simulink model "Static_pFIR"  (R2019b)
settings: Solver=FixedStepAuto  StartTime=0.0  StopTime=stop_time  RelTol=1e-3  EnableMultiTasking=on
InitFcn:
  | sm_callback_init
undefined symbols (not defined in the file or in its folder): a, b, B_k_0_init, c, FIR_0_Size, FIR_0_Uprate, Ts
libraries: simulink x10, hdlsllib x2
settings Model: Creator=Balad  LastModifiedBy=cb54103
settings DataIOCC: SaveOutput=off  SaveTime=off
settings OptimizationCC: BlockReduction=off  ConditionallyExecuteInputs=off  DefaultParameterBehavior=Inlined
settings DebuggingCC: SingleTaskRateTransMsg=error
settings SFSimCC: CustomCodeUndefinedFunction=UseInterfaceOnly

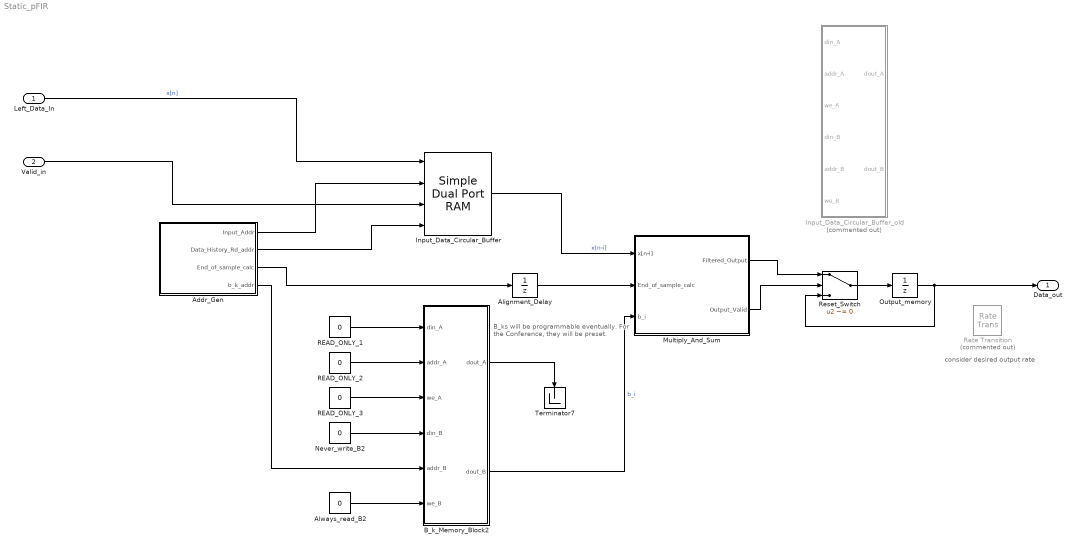
== system Static_pFIR ==
  note: consider desired output rate
  note: B_ks will be programmable eventually.
      | For the Conference, they will be preset.
  Left_Data_In : Inport  OutDataTypeStr=fixdt(1,32,28)  PortDimensions=[1 1]  SampleTime=[2.0345052083333333e-08,0]
  Valid_in : Inport  Port=2  OutDataTypeStr=boolean  PortDimensions=[1 1]  SampleTime=[2.0345052083333333e-08,0]
  "Addr_Gen " : Subsystem
  Alignment_Delay : UnitDelay  SampleTime=-1  HasFrameUpgradeWarning=on
  Always_read_B2 : Constant  Value=0  OutDataTypeStr=boolean  SampleTime=Ts/FIR_0_Uprate
  B_k_Memory_Block2 : Subsystem  AncestorBlock=DualPortRam_UNLOCKED/Dual Rate Dual Port RAM1  mask(Dual-rate dual-port RAM){ram_size=FIR_0_Size}
      mask prompts: ram_size "Address port width (2 to 28 bits)"
      mask help: This block simulates a dual-clock dual-port RAM with two data output ports.
      mask init:
      | hdlblkmask_drdpram();
      mask Help: helpview([docroot '/simulink/helptargets.map'],'HDL_dual_rate_dual_port_ram');
  Input_Data_Circular_Buffer : hdlsllib/HDL RAMs/Simple Dual Port RAM  ram_size=FIR_0_Size
      settings: SourceProductName=Simulink  SourceProductBaseCode=SL
  Input_Data_Circular_Buffer_old : Subsystem  Commented=on  AncestorBlock=DualPortRam_UNLOCKED/Dual Rate Dual Port RAM1  mask(Dual-rate dual-port RAM){ram_size=FIR_0_Size}
      mask prompts: ram_size "Address port width (2 to 28 bits)"
      mask help: This block simulates a dual-clock dual-port RAM with two data output ports.
      mask init:
      | hdlblkmask_drdpram();
      mask Help: helpview([docroot '/simulink/helptargets.map'],'HDL_dual_rate_dual_port_ram');
  Multiply_And_Sum : Subsystem
  Never_write_B2 : Constant  Value=0  OutDataTypeStr=fixdt(1,W_bits, F_bits)  SampleTime=Ts/FIR_0_Uprate
  Output_memory : UnitDelay  SampleTime=-1  HasFrameUpgradeWarning=on
  READ_ONLY_1 : Constant  Value=0  OutDataTypeStr=fixdt(1,W_bits, F_bits)  SampleTime=Ts/FIR_0_Uprate
  READ_ONLY_2 : Constant  Value=0  OutDataTypeStr=fixdt(0,FIR_0_Size, 0)  SampleTime=Ts/FIR_0_Uprate
  READ_ONLY_3 : Constant  Value=0  OutDataTypeStr=boolean  SampleTime=Ts/FIR_0_Uprate
  Rate Transition : RateTransition  Commented=on  OutPortSampleTime=Ts
  Reset_Switch : Switch  Criteria=u2 ~= 0
  Terminator7 : Terminator
  Data_out : Outport  OutDataTypeStr=fixdt(1,32,28)  PortDimensions=1  SampleTime=[2.0345052083333333e-08,0]  VectorParamsAs1DForOutWhenUnconnected=off
  wires:
  READ_ONLY_2/1 -> B_k_Memory_Block2/2(addr_A)
  Always_read_B2/1 -> B_k_Memory_Block2/6(we_B)
  B_k_Memory_Block2/1(dout_A) -> Terminator7/1
  "Addr_Gen "/3(End_of_sample_calc) -> Alignment_Delay/1
  B_k_Memory_Block2/2(dout_B) -> Multiply_And_Sum/3(b_i)  "b_i"
  Reset_Switch/1 -> Output_memory/1
  Multiply_And_Sum/2(Output_Valid) -> Reset_Switch/2
  READ_ONLY_1/1 -> B_k_Memory_Block2/1(din_A)
  Never_write_B2/1 -> B_k_Memory_Block2/4(din_B)
  Input_Data_Circular_Buffer/1 -> Multiply_And_Sum/1(x[n-i])  "x[n-i]"
  "Addr_Gen "/2(Data_History_Rd_addr) -> Input_Data_Circular_Buffer/4
  Valid_in/1 -> Input_Data_Circular_Buffer/3
  Output_memory/1 -> Reset_Switch/3, Data_out/1
  READ_ONLY_3/1 -> B_k_Memory_Block2/3(we_A)
  "Addr_Gen "/1(Input_Addr) -> Input_Data_Circular_Buffer/2
  Multiply_And_Sum/1(Filtered_Output) -> Reset_Switch/1
  "Addr_Gen "/4(b_k_addr) -> B_k_Memory_Block2/5(addr_B)
  Left_Data_In/1 -> Input_Data_Circular_Buffer/1  "x[n]"
  Alignment_Delay/1 -> Multiply_And_Sum/2(End_of_sample_calc)

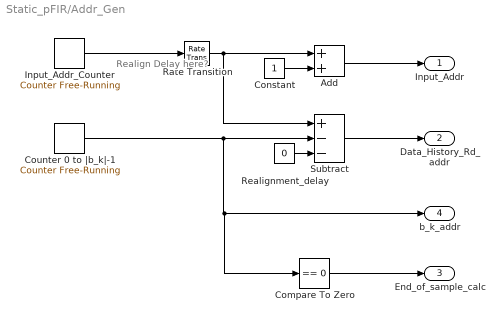
== system Static_pFIR/Addr_Gen  ==
  note: Realign Delay here?
  Add : Sum  OutDataTypeStr=Inherit: Same as first input
  Compare To Zero : simulink/Logic and Bit Operations/Compare To Zero  relop===  OutDataTypeStr=boolean  ZeroCross=off
  Constant : Constant  OutDataTypeStr=fixdt(0, FIR_0_Size,0)  SampleTime=-1
  Counter 0 to |b_k|-1 : simulink/Sources/Counter Free-Running  NumBits=FIR_0_Size  tsamp=Ts/FIR_0_Uprate
  Input_Addr_Counter : simulink/Sources/Counter Free-Running  NumBits=FIR_0_Size  tsamp=Ts
  Rate Transition : RateTransition  OutPortSampleTime=Ts/FIR_0_Uprate
  Realignment_delay : Constant  Value=0  OutDataTypeStr=fixdt(0, FIR_0_Size,0)  SampleTime=-1
  Subtract : Sum  Inputs=+--  OutDataTypeStr=Inherit: Same as first input
  Input_Addr : Outport  VectorParamsAs1DForOutWhenUnconnected=off
  Data_History_Rd_addr : Outport  Port=2  VectorParamsAs1DForOutWhenUnconnected=off
  End_of_sample_calc : Outport  Port=3  VectorParamsAs1DForOutWhenUnconnected=off
  b_k_addr : Outport  Port=4  VectorParamsAs1DForOutWhenUnconnected=off
  wires:
  Rate Transition/1 -> Add/1, Subtract/1
  Compare To Zero/1 -> End_of_sample_calc/1
  Realignment_delay/1 -> Subtract/3
  Constant/1 -> Add/2
  Add/1 -> Input_Addr/1
  Input_Addr_Counter/1 -> Rate Transition/1
  Subtract/1 -> Data_History_Rd_addr/1
  Counter 0 to |b_k|-1/1 -> b_k_addr/1, Compare To Zero/1, Subtract/2

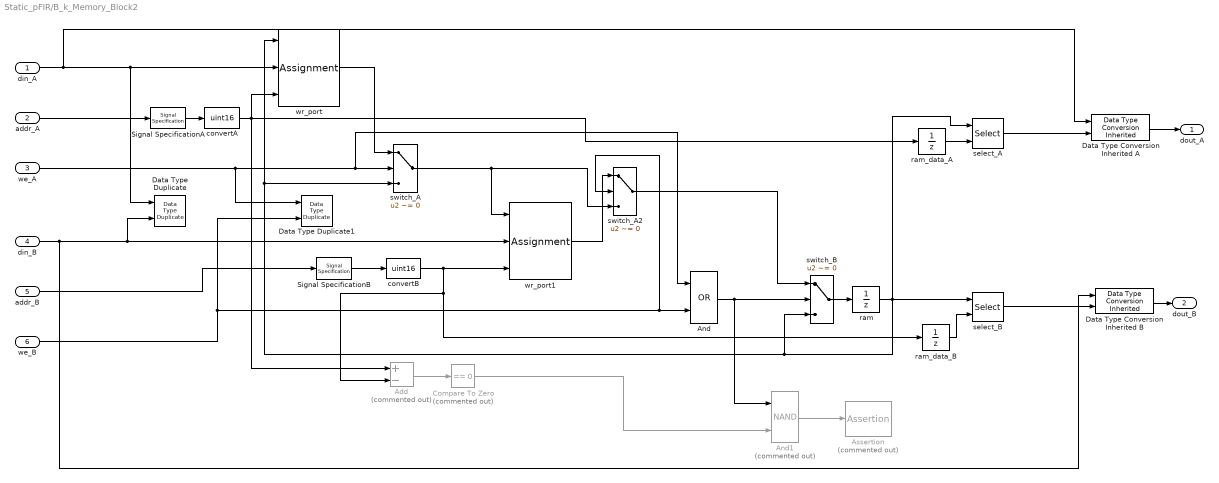
== system Static_pFIR/B_k_Memory_Block2 ==
  din_A : Inport
  addr_A : Inport  Port=2
  we_A : Inport  Port=3  OutDataTypeStr=boolean
  din_B : Inport  Port=4
  addr_B : Inport  Port=5
  we_B : Inport  Port=6  OutDataTypeStr=boolean
  Add : Sum  Commented=on  Inputs=+-
  And : Logic  Operator=OR  AllPortsSameDT=off  OutDataTypeStr=boolean
  And1 : Logic  Commented=on  Operator=NAND  AllPortsSameDT=off  OutDataTypeStr=boolean
  Assertion : Assertion  Commented=on  StopWhenAssertionFail=off
  Compare To Zero : simulink/Logic and Bit Operations/Compare To Zero  Commented=on  relop===  OutDataTypeStr=boolean
  Data Type Conversion Inherited A : simulink/Signal Attributes/Data Type Conversion Inherited  ConvertRealWorld=Real World Value  DoSatur=off
      settings: SourceProductName=Simulink  SourceProductBaseCode=SL
  Data Type Conversion Inherited B : simulink/Signal Attributes/Data Type Conversion Inherited  ConvertRealWorld=Real World Value  DoSatur=off
      settings: SourceProductName=Simulink  SourceProductBaseCode=SL
  Data Type Duplicate : DataTypeDuplicate
  Data Type Duplicate1 : DataTypeDuplicate
  Signal SpecificationA : SignalSpecification  OutDataTypeStr=fixdt(0,ram_size,0)  Dimensions=1
  Signal SpecificationB : SignalSpecification  OutDataTypeStr=fixdt(0,ram_size,0)  Dimensions=1
  convertA : DataTypeConversion  OutDataTypeStr=uint16
  convertB : DataTypeConversion  OutDataTypeStr=uint16
  ram : UnitDelay  InitialCondition=B_k_0_init  SampleTime=-1  HasFrameUpgradeWarning=on
  ram_data_A : UnitDelay  SampleTime=-1  HasFrameUpgradeWarning=on
  ram_data_B : UnitDelay  SampleTime=-1  HasFrameUpgradeWarning=on
  select_A : Selector  IndexMode=Zero-based  InputPortWidth=2^ram_size  IndexOptions=Index vector (port)  Indices=[1 3]  OutputSizes=1
  select_B : Selector  IndexMode=Zero-based  InputPortWidth=2^ram_size  IndexOptions=Index vector (port)  Indices=[1 3]  OutputSizes=1
  switch_A : Switch  Criteria=u2 ~= 0
  switch_A2 : Switch  Criteria=u2 ~= 0
  switch_B : Switch  Criteria=u2 ~= 0
  wr_port : Assignment  IndexMode=Zero-based  IndexOptions=Index vector (port)  Indices=1  OutputSizes=[1 1]
  wr_port1 : Assignment  IndexMode=Zero-based  IndexOptions=Index vector (port)  Indices=1  OutputSizes=[1 1]
  dout_A : Outport  VectorParamsAs1DForOutWhenUnconnected=off
  dout_B : Outport  Port=2  VectorParamsAs1DForOutWhenUnconnected=off
  wires:
  Data Type Conversion Inherited A/1 -> dout_A/1
  select_A/1 -> Data Type Conversion Inherited A/2
  Data Type Conversion Inherited B/1 -> dout_B/1
  select_B/1 -> Data Type Conversion Inherited B/2
  addr_A/1 -> Signal SpecificationA/1
  din_B/1 -> Data Type Conversion Inherited B/1, Data Type Duplicate/2, wr_port1/2
  convertB/1 -> wr_port1/3, Add/2, ram_data_B/1
  din_A/1 -> Data Type Conversion Inherited A/1, wr_port/2, Data Type Duplicate/1
  ram_data_A/1 -> select_A/2
  we_A/1 -> switch_A/2, And/1, Data Type Duplicate1/1
  ram_data_B/1 -> select_B/2
  addr_B/1 -> Signal SpecificationB/1
  switch_A/1 -> switch_A2/3, wr_port1/1
  we_B/1 -> Data Type Duplicate1/2, And/2, switch_A2/2
  Compare To Zero/1 -> And1/2
  Add/1 -> Compare To Zero/1
  wr_port1/1 -> switch_A2/1
  And/1 -> switch_B/2, And1/1
  wr_port/1 -> switch_A/1
  ram/1 -> select_A/1, wr_port/1, switch_A/3, switch_B/3, select_B/1
  convertA/1 -> Add/1, wr_port/3, ram_data_A/1
  switch_B/1 -> ram/1
  Signal SpecificationB/1 -> convertB/1
  Signal SpecificationA/1 -> convertA/1
  And1/1 -> Assertion/1
  switch_A2/1 -> switch_B/1

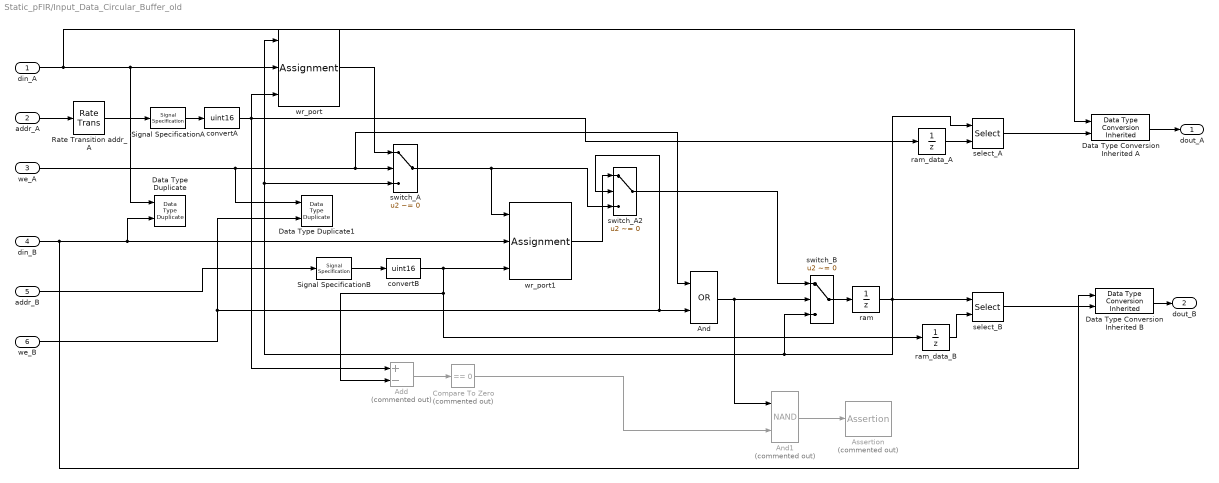
== system Static_pFIR/Input_Data_Circular_Buffer_old ==
  din_A : Inport
  addr_A : Inport  Port=2
  we_A : Inport  Port=3  OutDataTypeStr=boolean
  din_B : Inport  Port=4
  addr_B : Inport  Port=5
  we_B : Inport  Port=6  OutDataTypeStr=boolean
  Add : Sum  Commented=on  Inputs=+-
  And : Logic  Operator=OR  AllPortsSameDT=off  OutDataTypeStr=boolean
  And1 : Logic  Commented=on  Operator=NAND  AllPortsSameDT=off  OutDataTypeStr=boolean
  Assertion : Assertion  Commented=on  StopWhenAssertionFail=off
  Compare To Zero : simulink/Logic and Bit Operations/Compare To Zero  Commented=on  relop===  OutDataTypeStr=boolean
  Data Type Conversion Inherited A : simulink/Signal Attributes/Data Type Conversion Inherited  ConvertRealWorld=Real World Value  DoSatur=off
      settings: SourceProductName=Simulink  SourceProductBaseCode=SL
  Data Type Conversion Inherited B : simulink/Signal Attributes/Data Type Conversion Inherited  ConvertRealWorld=Real World Value  DoSatur=off
      settings: SourceProductName=Simulink  SourceProductBaseCode=SL
  Data Type Duplicate : DataTypeDuplicate
  Data Type Duplicate1 : DataTypeDuplicate
  Rate Transition addr_A : RateTransition
  Signal SpecificationA : SignalSpecification  OutDataTypeStr=fixdt(0,ram_size,0)  Dimensions=1
  Signal SpecificationB : SignalSpecification  OutDataTypeStr=fixdt(0,ram_size,0)  Dimensions=1
  convertA : DataTypeConversion  OutDataTypeStr=uint16
  convertB : DataTypeConversion  OutDataTypeStr=uint16
  ram : UnitDelay  SampleTime=-1  HasFrameUpgradeWarning=on
  ram_data_A : UnitDelay  SampleTime=-1  HasFrameUpgradeWarning=on
  ram_data_B : UnitDelay  SampleTime=-1  HasFrameUpgradeWarning=on
  select_A : Selector  IndexMode=Zero-based  InputPortWidth=2^ram_size  IndexOptions=Index vector (port)  Indices=[1 3]  OutputSizes=1
  select_B : Selector  IndexMode=Zero-based  InputPortWidth=2^ram_size  IndexOptions=Index vector (port)  Indices=[1 3]  OutputSizes=1
  switch_A : Switch  Criteria=u2 ~= 0
  switch_A2 : Switch  Criteria=u2 ~= 0
  switch_B : Switch  Criteria=u2 ~= 0
  wr_port : Assignment  IndexMode=Zero-based  IndexOptions=Index vector (port)  Indices=1  OutputSizes=[1 1]
  wr_port1 : Assignment  IndexMode=Zero-based  IndexOptions=Index vector (port)  Indices=1  OutputSizes=[1 1]
  dout_A : Outport  VectorParamsAs1DForOutWhenUnconnected=off
  dout_B : Outport  Port=2  VectorParamsAs1DForOutWhenUnconnected=off
  wires:
  switch_A2/1 -> switch_B/1
  And1/1 -> Assertion/1
  Signal SpecificationA/1 -> convertA/1
  Signal SpecificationB/1 -> convertB/1
  switch_B/1 -> ram/1
  convertA/1 -> ram_data_A/1, wr_port/3, Add/1
  ram/1 -> select_B/1, switch_B/3, switch_A/3, wr_port/1, select_A/1
  wr_port/1 -> switch_A/1
  And/1 -> And1/1, switch_B/2
  wr_port1/1 -> switch_A2/1
  Add/1 -> Compare To Zero/1
  Compare To Zero/1 -> And1/2
  we_B/1 -> switch_A2/2, And/2, Data Type Duplicate1/2
  switch_A/1 -> wr_port1/1, switch_A2/3
  addr_B/1 -> Signal SpecificationB/1
  ram_data_B/1 -> select_B/2
  we_A/1 -> Data Type Duplicate1/1, And/1, switch_A/2
  ram_data_A/1 -> select_A/2
  din_A/1 -> Data Type Conversion Inherited A/1, Data Type Duplicate/1, wr_port/2
  convertB/1 -> ram_data_B/1, Add/2, wr_port1/3
  din_B/1 -> Data Type Conversion Inherited B/1, wr_port1/2, Data Type Duplicate/2
  addr_A/1 -> Rate Transition addr_A/1
  Rate Transition addr_A/1 -> Signal SpecificationA/1
  select_B/1 -> Data Type Conversion Inherited B/2
  Data Type Conversion Inherited B/1 -> dout_B/1
  select_A/1 -> Data Type Conversion Inherited A/2
  Data Type Conversion Inherited A/1 -> dout_A/1

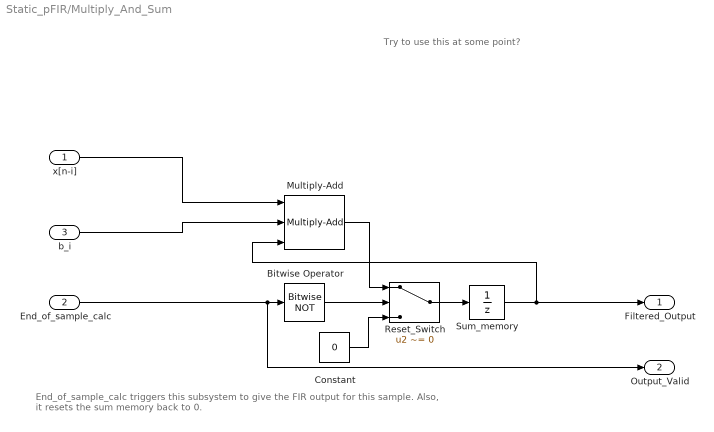
== system Static_pFIR/Multiply_And_Sum ==
  note: End_of_sample_calc triggers this subsystem to give the FIR output for this sample.
      | Also, it resets the sum memory back to 0.
  note: Try to use this at some point?
  x[n-i] : Inport
  End_of_sample_calc : Inport  Port=2
  b_i : Inport  Port=3
  Bitwise Operator : simulink/Logic and Bit Operations/Bitwise Operator  logicop=NOT  UseBitMask=off  BitMask=bin2dec('11011001')  BitMaskRealWorld=Stored Integer
  Constant : Constant  Value=0  OutDataTypeStr=fixdt(1, W_bits, F_bits)  SampleTime=Ts/FIR_0_Uprate
  Multiply-Add : hdlsllib/HDL Operations/Multiply-Add  Function=c+(a.*b)  datatype=Inherit: Same as first input  DoSatur=off  FMA=off
      settings: SourceProductName=Simulink  SourceProductBaseCode=SL
  Reset_Switch : Switch  Criteria=u2 ~= 0  ZeroCross=off
  Sum_memory : UnitDelay  SampleTime=-1  HasFrameUpgradeWarning=on
  Filtered_Output : Outport  VectorParamsAs1DForOutWhenUnconnected=off
  Output_Valid : Outport  Port=2  VectorParamsAs1DForOutWhenUnconnected=off
  wires:
  Bitwise Operator/1 -> Reset_Switch/2
  Constant/1 -> Reset_Switch/3
  Reset_Switch/1 -> Sum_memory/1
  Multiply-Add/1 -> Reset_Switch/1
  Sum_memory/1 -> Filtered_Output/1, Multiply-Add/3
  b_i/1 -> Multiply-Add/2
  End_of_sample_calc/1 -> Bitwise Operator/1, Output_Valid/1
  x[n-i]/1 -> Multiply-Add/1
